simulink model "simulink_2_balloons"  (R2020b)
settings: Solver=VariableStepAuto  StartTime=0.0  StopTime=300  RelTol=1e-3
InitFcn:
  | seed1 = randi(100000);
  | seed2 = randi(200000);
values from neighbouring files (symbols this model uses):
  Cd = 0.185    [sim_1balloon.m]    (also in sim_1balloon_test.m; sim_2balloon.m; sim_2balloon_test.m; sim_4balloon.m)
  coefficient_dragq = [-0.285 -0.20532562963 -0.122209481481 -0.036512 0.0509063703704 0.139185185185 0.227464 0.31488237037 0.400579851852 0.483696 0.56337037037 0.638742518519 ... (72581 elements, 181x401)]    [coefficient_dragq.mat]
  coefficient_sideforceq = [0 -0.0269042962963 -0.0553588148148 -0.084976 -0.115368296296 -0.146148148148 -0.176928 -0.207320296296 -0.236937481481 -0.265392 -0.292296296296 -0.317262814815 ... (72581 elements, 181x401)]    [coefficient_sideforceq.mat]
  mb1 = 3/1000    (= 0.003)    [sim_1balloon.m]    (also in sim_1balloon_test.m; sim_2balloon.m; sim_2balloon_test.m; sim_4balloon.m)
  mb2 = 3/1000    (= 0.003)    [sim_2balloon.m]    (also in sim_2balloon_test.m; sim_4balloon.m; sim_4balloon_test.m)
  nH = optimizableVariable('nH',nHB)    [optimiseB2.m]    (also in optimiseB4.m; sim_1balloon.m = x(2); sim_1balloon_test.m = x(2); sim_2balloon.m = x(2))
  normalScaling = optimizableVariable('normalScaling',normalScalingB)    [optimiseB2.m]    (also in optimiseB4.m; sim_1balloon.m = x(5); sim_1balloon_test.m = x(5); sim_2balloon.m = x(5))
  nS = optimizableVariable('nS',nSB)    [optimiseB2.m]    (also in optimiseB4.m; sim_1balloon.m = x(3); sim_1balloon_test.m = x(3); sim_2balloon.m = x(3))
  nV = optimizableVariable('nV',nVB)    [optimiseB2.m]    (also in optimiseB4.m; sim_1balloon.m = x(1); sim_1balloon_test.m = x(1); sim_2balloon.m = x(1))
  rb = 80/1000    (= 0.08)    [sim_1balloon.m]    (also in sim_1balloon_test.m; sim_2balloon.m; sim_2balloon_test.m; sim_4balloon.m)
  rb1 = 80/1000    (= 0.08)    [sim_1balloon.m]    (also in sim_1balloon_test.m; sim_2balloon.m; sim_2balloon_test.m; sim_4balloon.m)
  rb2 = 80/1000    (= 0.08)    [sim_2balloon.m]    (also in sim_2balloon_test.m; sim_4balloon.m; sim_4balloon_test.m)
  rn = 125/2000    (= 0.0625)    [sim_1balloon.m]    (also in sim_1balloon_test.m; sim_2balloon.m; sim_2balloon_test.m; sim_4balloon.m)
  seedX1 = randi(100000)    [sim_1balloon.m]    (also in sim_1balloon_test.m = x(8); sim_2balloon.m; sim_2balloon_test.m = x(11); sim_4balloon.m)
  seedX2 = randi(100000)    [sim_2balloon.m]    (also in sim_2balloon_test.m = x(14); sim_4balloon.m; sim_4balloon_test.m = x(14))
  seedY1 = randi(100000)    [sim_1balloon.m]    (also in sim_1balloon_test.m = x(9); sim_2balloon.m; sim_2balloon_test.m = x(12); sim_4balloon.m)
  seedY2 = randi(100000)    [sim_2balloon.m]    (also in sim_2balloon_test.m = x(15); sim_4balloon.m; sim_4balloon_test.m = x(15))
  seedZ1 = randi(100000)    [sim_1balloon.m]    (also in sim_1balloon_test.m = x(10); sim_2balloon.m; sim_2balloon_test.m = x(13); sim_4balloon.m)
  seedZ2 = randi(100000)    [sim_2balloon.m]    (also in sim_2balloon_test.m = x(16); sim_4balloon.m; sim_4balloon_test.m = x(16))
  theta = optimizableVariable('theta',thetaB)    [optimiseB2.m]    (also in optimiseB4.m; sim_1balloon.m = x(7); sim_1balloon_test.m = x(7); sim_2balloon.m = x(7))
  V0 = optimizableVariable('V0',V0B)    [optimiseB1.m]    (also in optimiseB2.m; optimiseB4.m; sim_1balloon.m = x(4); sim_1balloon_test.m = x(4))
libraries: nesl_utility x21, sm_lib x12, eeGeneralControl x6
settings Model: Creator=toby  LastModifiedBy=dante
settings ExplorerConfigSet: InternalSimMechanicsExplorerSettings="<ExplorerConfiguration><canonicalview>default</canonicalview><AnimationSetting><BasePlaybackSpeed>1.0</BasePlaybackSpeed><PlaybackSpeedFactor>1.0</PlaybackSpeedFactor></AnimationSetting><TilePanel><TileInfo><Tiles Columns=\"1\" Count=\"1\" Rows=\"1\"><Column Weight=\"1\"/><Row Weight=\"1\"/><Tile Height=\"1\" Width=\"1\" X=\"0\" Y=\"0\"/></Tiles></TileInfo><SceneInfo><SceneViewer><BGColor><R>0.60000002384185791</R><G>0.60000002384185791</G><B>0.60000002384185791</B></BGColor><Camera><DoPerspective>off</DoPerspective><Position><X>-0.0428873579630689797</X><Y>-0.981698513031005859</Y><Z>0.930594914501606474</Z></Position><Center><X>-0.0428873579630689797</X><Y>0.0183014869689941406</Y><Z>0.930594914501606474</Z></Center><Up><X>0</X><Y>-0</Y><Z>1</Z></Up><ViewLimDist>1</ViewLimDist><YLim>0.975489363470708692</YLim><XLim>1.38819640186216242</XLim></Camera></SceneViewer></SceneInfo></TilePanel><MechEditorPanel><Cameras/><GfxPanelCameraMap/><VideoCreator><PlaybackSpeedRatio>1.0</PlaybackSpeedRatio><FrameRate>30</FrameRate><VideoFormat>MPEG-4</VideoFormat><FrameSize>auto</FrameSize></VideoCreator></MechEditorPanel></ExplorerConfiguration>"

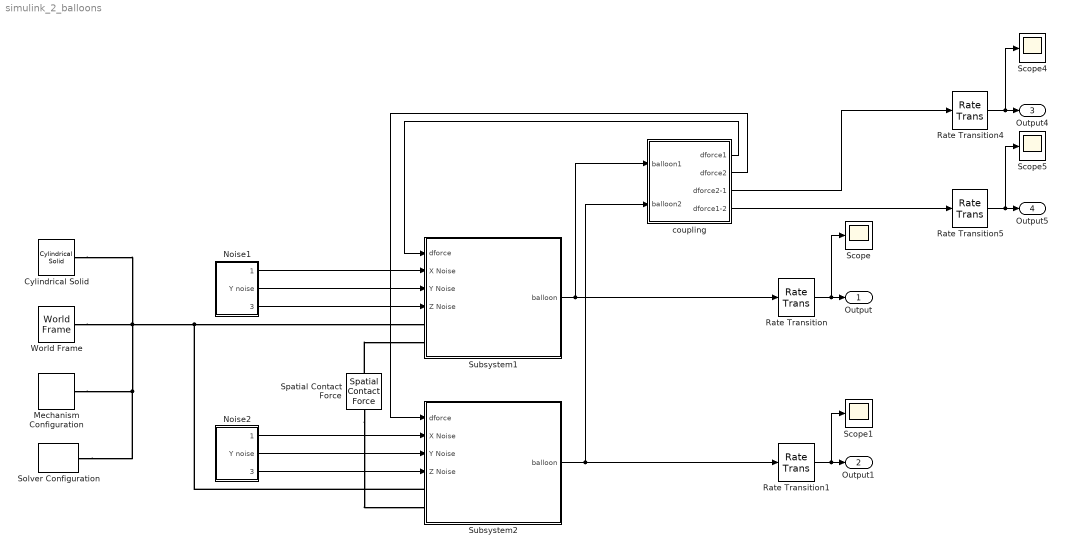
== system simulink_2_balloons ==
  Cylindrical Solid : sm_lib/Body Elements/Cylindrical Solid  GraphicAmbientColor=[0.15 0.15 0.15 1.0]  BasedOnType=Density  CenterOfMass=[0 0 0]  CenterOfMassUnits=m  GraphicDiffuseColor=[0.2 1.0 1.0]  CylinderLength=0.01  CylinderLengthUnits=m  CylinderRadius=rn  CylinderRadiusUnits=m  Density=1000  DensityUnits=kg/m^3  DoExposeReferenceFrame=on  GraphicEmissiveColor=[0.0 0.0 0.0 1.0]  ExportEntireGeometry=off  SerializedFrames=<Frames/>  MarkerShape=Sphere  MarkerSize=10  GraphicType=FromGeometry  InertiaType=CalculateFromGeometry  Mass=1  MassUnits=kg  MomentsOfInertia=[1 1 1]  MomentsOfInertiaUnits=kg*m^2  GraphicOpacity=1.0  ProductsOfInertia=[0 0 0]  ProductsOfInertiaUnits=kg*m^2  GraphicShininess=75  GraphicSpecularColor=[0.5 0.5 0.5 1.0]  GraphicVisPropType=SimpleVisualProperties
  Mechanism Configuration : sm_lib/Utilities/Mechanism Configuration  UniformGravity=Constant  GravityVector=[0 0 -9.81]  GravityVectorUnits=m/s^2  GravityUnits=m/s^2  LinearizationDelta=0.001  JointModeTransitionNonlinearIterations=2
  Noise1 : Subsystem
  Noise2 : Subsystem
  Rate Transition{,1,4..5} (4 alike) : RateTransition  OutPortSampleTime=1/30
  Scope{,1,4..5} (4 alike) : Scope
  Solver Configuration : nesl_utility/Solver Configuration  PhysicalDomain=network_engine_domain  SubClassName=solver  LeftPortType=input  RightPortType=generic  Tones=[]  Harmonics=[]  SimulateNoise=off  Profile=off  UseLocalSampling=off  EnableSwitchedLinearOptims=on  FrequencyDomain=off  UseCCode=off  RelTol=0.001  AbsTol=1e-06  MinStep=1e-09  ToWorkspace=off  RevertToSquareIcSolve=off  NumHomotopyIterations=100  PhasorMode=off  PhasorModeNumHarmonics=1  DoDC=off  ResidualTolerance=1e-9  UseLocalSolver=off  LocalSolverChoice=NE_BACKWARD_EULER_ADVANCER  LocalSolverSampleTime=.001  DoFixedCost=off  MaxNonlinIter=3  MaxModeIter=2  ComputeImpulses=off  ImpulseIterations=2  LinearAlgebra=Sparse  EquationFormulation=NE_TIME_EF  DelaysMemoryBudget=1024  AutomaticFiltering=on  FilteringTimeConstant=0.001  PartitionStorageMethod=AS_NEEDED  PartitionMemoryBudget=1024  PartitionMethod=FAST
  Spatial Contact Force : sm_lib/Forces and Torques/Spatial Contact Force  CoefficientOfDynamicFriction=0.1  CoefficientOfStaticFriction=0.1  NormalDamping=d  NormalDampingUnits=N/(m/s)  NormalStiffness=k  NormalStiffnessUnits=N/m  FrictionalCriticalVelocity=1e-3  FrictionalCriticalVelocityUnits=m/s  ZeroCrossDetectContactStartAndEnd=off  SenseFrictionalForceMagnitude=off  SenseNormalForceMagnitude=off  SenseSeparationDistance=off  NormalTransitionRegionWidth=tw  NormalTransitionRegionWidthUnits=m  FrictionType=SmoothStickSlip
  Subsystem1 : Subsystem  mask{initialHeight=0.2, ix=0, iy=0, balloonRadius=rb1, balloonMass=mb1, nozzleRadius=rn, theta=theta, V0=V0, Cd=Cd, normalScaling=normalScaling}
      mask prompts: initialHeight "initial height"; balloonRadius "balloon radius"; balloonMass "balloon mass"
  Subsystem2 : Subsystem  mask{initialHeight=0.4, ix=0, iy=0, balloonRadius=rb2, balloonMass=mb2, nozzleRadius=rn, theta=theta, V0=V0, Cd=Cd, normalScaling=normalScaling}
      mask prompts: initialHeight "initial height"; balloonRadius "balloon radius"; balloonMass "balloon mass"
  World Frame : sm_lib/Frames and Transforms/World Frame
  coupling : Subsystem
  Output : Outport
  Output1 : Outport  Port=2
  Output4 : Outport  Port=3
  Output5 : Outport  Port=4
  wires:
  Noise1/1(X noise) -> Subsystem1/2(X Noise)
  Rate Transition/1 -> Scope/1, Output/1
  Noise1/3(Z noise) -> Subsystem1/4(Z Noise)
  Noise1/2(" Y noise") -> Subsystem1/3(Y Noise)
  Rate Transition1/1 -> Scope1/1, Output1/1
  Noise2/3(Z noise) -> Subsystem2/4(Z Noise)
  Noise2/2(" Y noise") -> Subsystem2/3(Y Noise)
  Noise2/1(X noise) -> Subsystem2/2(X Noise)
  Subsystem1/1(balloon) -> Rate Transition/1, coupling/1(balloon1)
  coupling/1(dforce1) -> Subsystem1/1(dforce)
  Subsystem2/1(balloon) -> Rate Transition1/1, coupling/2(balloon2)
  coupling/2(dforce2) -> Subsystem2/1(dforce)
  Rate Transition4/1 -> Scope4/1, Output4/1
  Rate Transition5/1 -> Scope5/1, Output5/1
  coupling/3(dforce2-1) -> Rate Transition4/1
  coupling/4(dforce1-2) -> Rate Transition5/1
  connections:
  World Frame/RConn1 -- Solver Configuration/RConn1 -- Mechanism Configuration/RConn1 -- Subsystem2/LConn1 -- Subsystem1/LConn1 -- Cylindrical Solid/RConn1
  Spatial Contact Force/LConn1 -- Subsystem1/LConn2
  Spatial Contact Force/RConn1 -- Subsystem2/LConn2

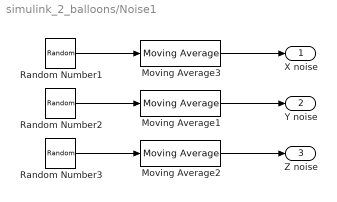
== system simulink_2_balloons/Noise1 ==
  Moving Average1 : eeGeneralControl/Moving Average  VariantControl=Variant1  LabelModeActiveChoice=Discrete  f=10  x0=0  Ts=nS/10
      settings: SourceProductBaseCode=PS
  Moving Average2 : eeGeneralControl/Moving Average  VariantControl=Variant1  LabelModeActiveChoice=Discrete  f=10  x0=0  Ts=nS/10
      settings: SourceProductBaseCode=PS
  Moving Average3 : eeGeneralControl/Moving Average  VariantControl=Variant1  LabelModeActiveChoice=Discrete  f=10  x0=0  Ts=nS/10
      settings: SourceProductBaseCode=PS
  Random Number1 : RandomNumber  Variance=nH  Seed=seedX1  SampleTime=nS
  Random Number2 : RandomNumber  Variance=nH  Seed=seedY1  SampleTime=nS
  Random Number3 : RandomNumber  Variance=nV  Seed=seedZ1  SampleTime=nS
  X noise : Outport
  " Y noise" : Outport  Port=2
  Z noise : Outport  Port=3
  wires:
  Random Number2/1 -> Moving Average1/1
  Moving Average3/1 -> X noise/1
  Random Number3/1 -> Moving Average2/1
  Random Number1/1 -> Moving Average3/1
  Moving Average1/1 -> " Y noise"/1
  Moving Average2/1 -> Z noise/1

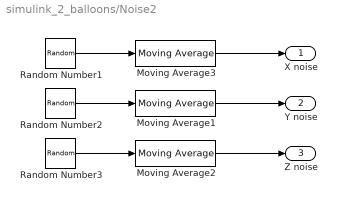
== system simulink_2_balloons/Noise2 ==
  Moving Average1 : eeGeneralControl/Moving Average  VariantControl=Variant1  LabelModeActiveChoice=Discrete  f=10  x0=0  Ts=nS/10
      settings: SourceProductBaseCode=PS
  Moving Average2 : eeGeneralControl/Moving Average  VariantControl=Variant1  LabelModeActiveChoice=Discrete  f=10  x0=0  Ts=nS/10
      settings: SourceProductBaseCode=PS
  Moving Average3 : eeGeneralControl/Moving Average  VariantControl=Variant1  LabelModeActiveChoice=Discrete  f=10  x0=0  Ts=nS/10
      settings: SourceProductBaseCode=PS
  Random Number1 : RandomNumber  Variance=nH  Seed=seedX2  SampleTime=nS
  Random Number2 : RandomNumber  Variance=nH  Seed=seedY2  SampleTime=nS
  Random Number3 : RandomNumber  Variance=nV  Seed=seedZ2  SampleTime=nS
  X noise : Outport
  " Y noise" : Outport  Port=2
  Z noise : Outport  Port=3
  wires:
  Random Number2/1 -> Moving Average1/1
  Moving Average3/1 -> X noise/1
  Random Number3/1 -> Moving Average2/1
  Random Number1/1 -> Moving Average3/1
  Moving Average1/1 -> " Y noise"/1
  Moving Average2/1 -> Z noise/1

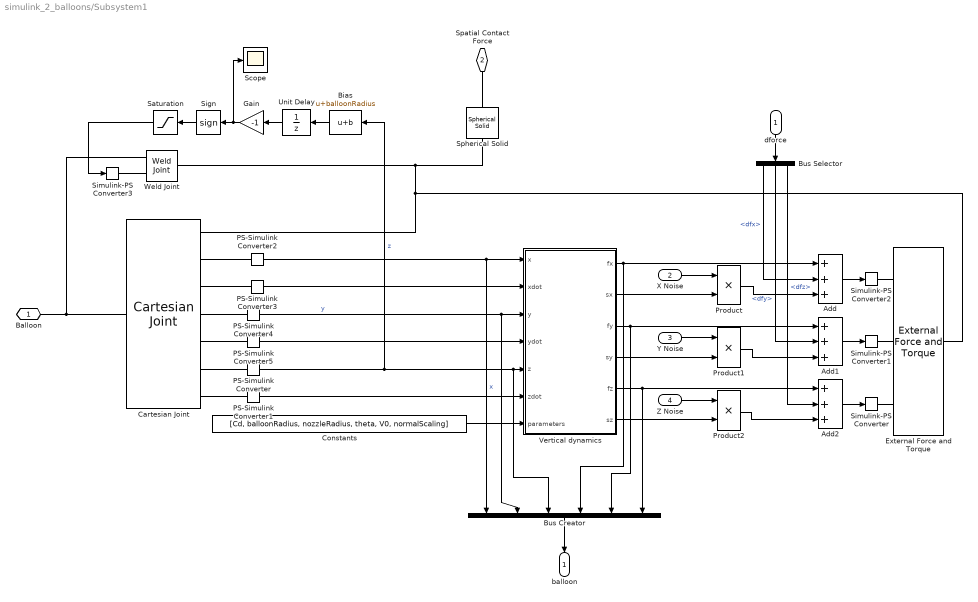
== system simulink_2_balloons/Subsystem1 ==
  dforce : Inport
  X Noise : Inport  Port=2
  Y Noise : Inport  Port=3
  Z Noise : Inport  Port=4
  Add : Sum  Inputs=+++
  Add1 : Sum  Inputs=+++
  Add2 : Sum  Inputs=+++
  Bias : Bias  Bias=balloonRadius
  Bus Creator : BusCreator  Inputs=6
  Bus Selector : BusSelector  OutputSignals=dfx,dfy,dfz
  Cartesian Joint : sm_lib/Joints/Cartesian Joint  JointMode=Normal  SenseConstraintForce=off  SenseConstraintForceX=off  SenseConstraintForceY=off  SenseConstraintForceZ=off  SenseConstraintTorque=off  SenseConstraintTorqueX=off  SenseConstraintTorqueY=off  SenseConstraintTorqueZ=off  SenseTotalForce=off  SenseTotalForceX=off  SenseTotalForceY=off  SenseTotalForceZ=off  SenseTotalTorque=off  SenseTotalTorqueX=off  SenseTotalTorqueY=off  SenseTotalTorqueZ=off  CompositeWrenchDir=FollowerOnBase  CompositeWrenchFrame=BaseFrame  PxEquilibriumPosition=0  PxEquilibriumPositionUnits=m  PxSpringStiffness=0  PxSpringStiffnessUnits=N/m  PxDampingCoefficient=hd  PxDampingCoefficientUnits=N/(m/s)  PxTorqueActuationMode=NoTorque  PxMotionActuationMode=ComputedMotion  PxSensePosition=on  PxSenseVelocity=on  PxSenseAcceleration=off  PxSenseTorqueForce=off  PxSenseLowerLimitTorqueForce=off  PxSenseUpperLimitTorqueForce=off  PxLowerLimitSpecify=off  PxLowerLimitBound=-1  PxLowerLimitBoundUnits=m  PxLowerLimitStiffness=1e6  PxLowerLimitStiffnessUnits=N/m  PxLowerLimitDamping=1e3  PxLowerLimitDampingUnits=N/(m/s)  PxLowerLimitTransitionRegionWidth=1e-4  PxLowerLimitTransitionRegionWidthUnits=m  PxUpperLimitSpecify=off  PxUpperLimitBound=1  PxUpperLimitBoundUnits=m  PxUpperLimitStiffness=1e6  PxUpperLimitStiffnessUnits=N/m  PxUpperLimitDamping=1e3  PxUpperLimitDampingUnits=N/(m/s)  PxUpperLimitTransitionRegionWidth=1e-4  PxUpperLimitTransitionRegionWidthUnits=m  PxPositionTargetSpecify=off  PxPositionTargetPriority=High  PxPositionTargetValue=0  PxPositionTargetValueUnits=m  PxVelocityTargetSpecify=off  PxVelocityTargetPriority=High  PxVelocityTargetValue=0  PxVelocityTargetValueUnits=m/s  PyEquilibriumPosition=0  PyEquilibriumPositionUnits=m  PySpringStiffness=0  PySpringStiffnessUnits=N/m  PyDampingCoefficient=hd  PyDampingCoefficientUnits=N/(m/s)  PyTorqueActuationMode=NoTorque  PyMotionActuationMode=ComputedMotion  PySensePosition=on  PySenseVelocity=on  PySenseAcceleration=off  PySenseTorqueForce=off  PySenseLowerLimitTorqueForce=off  PySenseUpperLimitTorqueForce=off  PyLowerLimitSpecify=off  PyLowerLimitBound=-1  PyLowerLimitBoundUnits=m  PyLowerLimitStiffness=1e6  PyLowerLimitStiffnessUnits=N/m  PyLowerLimitDamping=1e3  PyLowerLimitDampingUnits=N/(m/s)  PyLowerLimitTransitionRegionWidth=1e-4  PyLowerLimitTransitionRegionWidthUnits=m  PyUpperLimitSpecify=off  PyUpperLimitBound=1  PyUpperLimitBoundUnits=m  PyUpperLimitStiffness=1e6  PyUpperLimitStiffnessUnits=N/m  PyUpperLimitDamping=1e3  PyUpperLimitDampingUnits=N/(m/s)  PyUpperLimitTransitionRegionWidth=1e-4  PyUpperLimitTransitionRegionWidthUnits=m  PyPositionTargetSpecify=off  PyPositionTargetPriority=High  PyPositionTargetValue=0  PyPositionTargetValueUnits=m  PyVelocityTargetSpecify=off  PyVelocityTargetPriority=High  PyVelocityTargetValue=0  PyVelocityTargetValueUnits=m/s  PzEquilibriumPosition=0  PzEquilibriumPositionUnits=m  PzSpringStiffness=0  PzSpringStiffnessUnits=N/m  PzDampingCoefficient=hd  PzDampingCoefficientUnits=N/(m/s)  PzTorqueActuationMode=NoTorque  PzMotionActuationMode=ComputedMotion  PzSensePosition=on  PzSenseVelocity=on  PzSenseAcceleration=off  PzSenseTorqueForce=off  PzSenseLowerLimitTorqueForce=off  PzSenseUpperLimitTorqueForce=off  PzLowerLimitSpecify=off  PzLowerLimitBound=0  PzLowerLimitBoundUnits=m  PzLowerLimitStiffness=1e6  PzLowerLimitStiffnessUnits=N/m  PzLowerLimitDamping=1e3  PzLowerLimitDampingUnits=N/(m/s)  PzLowerLimitTransitionRegionWidth=1e-4  PzLowerLimitTransitionRegionWidthUnits=m  PzUpperLimitSpecify=off  PzUpperLimitBound=1  PzUpperLimitBoundUnits=m  PzUpperLimitStiffness=1e6  PzUpperLimitStiffnessUnits=N/m  PzUpperLimitDamping=1e3  PzUpperLimitDampingUnits=N/(m/s)  PzUpperLimitTransitionRegionWidth=1e-4  PzUpperLimitTransitionRegionWidthUnits=m  PzPositionTargetSpecify=on  PzPositionTargetPriority=High  PzPositionTargetValue=initialHeight  PzPositionTargetValueUnits=m  PzVelocityTargetSpecify=on  PzVelocityTargetPriority=High  PzVelocityTargetValue=0  PzVelocityTargetValueUnits=m/s
  Constants : Constant  Value=[Cd, balloonRadius, nozzleRadius, theta, V0, normalScaling]
  External Force and Torque : sm_lib/Forces and Torques/External Force and Torque  ForceResolutionFrame=AttachedFrame  EnableForceX=on  EnableForceY=on  EnableForceZ=on  EnableForce=off  TorqueResolutionFrame=AttachedFrame  EnableTorqueX=off  EnableTorqueY=off  EnableTorqueZ=off  EnableTorque=off
  Gain : Gain  Gain=-1
  PS-Simulink Converter{,1..5} (6 alike) : nesl_utility/PS-Simulink Converter  PhysicalDomain=network_engine_domain  SubClassName=ps_output  LeftPortType=input  RightPortType=output  PseudoPeriodic=off  Frequencies=[]  Unit=inherit  AffineConversion=off
  Product : Product
  Product1 : Product
  Product2 : Product
  Saturation : Saturate  UpperLimit=0  LowerLimit=-1
  Scope : Scope
  Sign : Signum
  Simulink-PS Converter{,1..3} (4 alike) : nesl_utility/Simulink-PS Converter  PhysicalDomain=network_engine_domain  SubClassName=ps_input  LeftPortType=input  RightPortType=output  PseudoPeriodic=off  Frequencies=[]  NoiseDistribution=none  NoiseParameters=[]  Unit=1  AffineConversion=off  FilteringAndDerivatives=provide  SimscapeFilterOrder=1  InputFilterTimeConstant=0.001  UdotUserProvided=0
  Spherical Solid : sm_lib/Body Elements/Spherical Solid  GraphicAmbientColor=[0.15 0.15 0.15 1.0]  BasedOnType=Mass  CenterOfMass=[0 0 0]  CenterOfMassUnits=m  GraphicDiffuseColor=[1.0 0.0 0.0]  Density=1000  DensityUnits=kg/m^3  DoExposeReferenceFrame=on  GraphicEmissiveColor=[0.0 0.0 0.0 1.0]  ExportEntireGeometry=on  SerializedExposedGeometries=<ExposedGeometries><ExposedGeometry><RawGeometryId>entire</RawGeometryId><ExposedGeometryId>G</ExposedGeometryId></ExposedGeometry></ExposedGeometries>  SerializedFrames=<Frames/>  MarkerShape=Sphere  MarkerSize=10  GraphicType=FromGeometry  InertiaType=CalculateFromGeometry  Mass=balloonMass  MassUnits=kg  MomentsOfInertia=[1 1 1]  MomentsOfInertiaUnits=kg*m^2  GraphicOpacity=1.0  ProductsOfInertia=[0 0 0]  ProductsOfInertiaUnits=kg*m^2  GraphicShininess=75  GraphicSpecularColor=[0.5 0.5 0.5 1.0]  SphereRadius=balloonRadius  SphereRadiusUnits=m  GraphicVisPropType=SimpleVisualProperties
  Unit Delay : UnitDelay  InitialCondition=initialHeight+balloonRadius  SampleTime=0.01  HasFrameUpgradeWarning=on
  Vertical dynamics : MATLAB Function  TreatAsAtomicUnit=on
  Weld Joint : sm_lib/Joints/Weld Joint  JointMode=ProvidedByInput  SenseConstraintForce=off  SenseConstraintForceX=off  SenseConstraintForceY=off  SenseConstraintForceZ=off  SenseConstraintTorque=off  SenseConstraintTorqueX=off  SenseConstraintTorqueY=off  SenseConstraintTorqueZ=off  SenseTotalForce=off  SenseTotalForceX=off  SenseTotalForceY=off  SenseTotalForceZ=off  SenseTotalTorque=off  SenseTotalTorqueX=off  SenseTotalTorqueY=off  SenseTotalTorqueZ=off  CompositeWrenchDir=FollowerOnBase  CompositeWrenchFrame=BaseFrame
  Balloon : PMIOPort  Side=Left
  Spatial Contact Force : PMIOPort  Port=2  Side=Left
  balloon : Outport
  wires:
  PS-Simulink Converter3/1 -> Vertical dynamics/2(xdot)
  PS-Simulink Converter4/1 -> Vertical dynamics/3(y), Bus Creator/2  "y"
  PS-Simulink Converter2/1 -> Vertical dynamics/1(x), Bus Creator/1  "x"
  PS-Simulink Converter5/1 -> Vertical dynamics/4(ydot)
  Constants/1 -> Vertical dynamics/7(parameters)
  PS-Simulink Converter/1 -> Bus Creator/3, Vertical dynamics/5(z), Bias/1  "z"
  PS-Simulink Converter1/1 -> Vertical dynamics/6(zdot)
  Vertical dynamics/2(sx) -> Product/2
  Vertical dynamics/4(sy) -> Product1/2
  Vertical dynamics/6(sz) -> Product2/2
  Gain/1 -> Scope/1, Sign/1
  Unit Delay/1 -> Gain/1
  Sign/1 -> Saturation/1
  Saturation/1 -> Simulink-PS Converter3/1
  Bias/1 -> Unit Delay/1
  Z Noise/1 -> Product2/1
  Add/1 -> Simulink-PS Converter2/1
  Add1/1 -> Simulink-PS Converter1/1
  Add2/1 -> Simulink-PS Converter/1
  Y Noise/1 -> Product1/1
  X Noise/1 -> Product/1
  Vertical dynamics/5(fz) -> Add2/1, Bus Creator/6
  Vertical dynamics/3(fy) -> Add1/1, Bus Creator/5
  Vertical dynamics/1(fx) -> Add/1, Bus Creator/4
  Bus Creator/1 -> balloon/1
  dforce/1 -> Bus Selector/1
  Product2/1 -> Add2/3
  Product1/1 -> Add1/3
  Product/1 -> Add/3
  Bus Selector/3 -> Add2/2  "<dfz>"
  Bus Selector/2 -> Add1/2  "<dfy>"
  Bus Selector/1 -> Add/2  "<dfx>"
  connections:
  PS-Simulink Converter/LConn1 -- Cartesian Joint/RConn6
  PS-Simulink Converter2/LConn1 -- Cartesian Joint/RConn2
  Weld Joint/RConn1 -- Spherical Solid/RConn1 -- Cartesian Joint/RConn1 -- External Force and Torque/RConn1
  Cartesian Joint/LConn1 -- Weld Joint/LConn1 -- Balloon/RConn1
  PS-Simulink Converter5/LConn1 -- Cartesian Joint/RConn5
  Simulink-PS Converter/RConn1 -- External Force and Torque/LConn3
  External Force and Torque/LConn1 -- Simulink-PS Converter2/RConn1
  Simulink-PS Converter1/RConn1 -- External Force and Torque/LConn2
  Cartesian Joint/RConn4 -- PS-Simulink Converter4/LConn1
  PS-Simulink Converter3/LConn1 -- Cartesian Joint/RConn3
  PS-Simulink Converter1/LConn1 -- Cartesian Joint/RConn7
  Simulink-PS Converter3/RConn1 -- Weld Joint/LConn2
  Spatial Contact Force/RConn1 -- Spherical Solid/LConn1

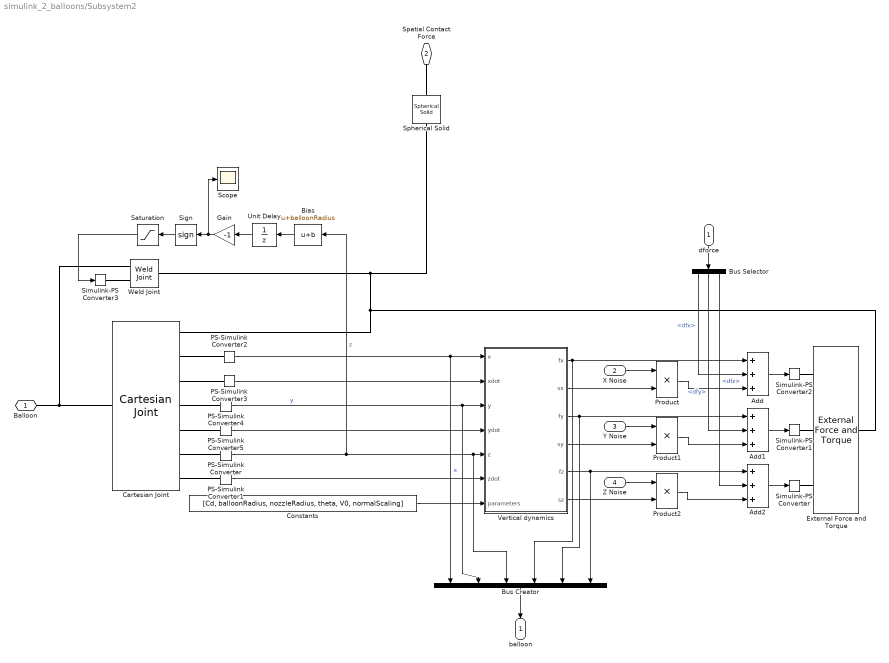
== system simulink_2_balloons/Subsystem2 ==
  dforce : Inport
  X Noise : Inport  Port=2
  Y Noise : Inport  Port=3
  Z Noise : Inport  Port=4
  Add : Sum  Inputs=+++
  Add1 : Sum  Inputs=+++
  Add2 : Sum  Inputs=+++
  Bias : Bias  Bias=balloonRadius
  Bus Creator : BusCreator  Inputs=6
  Bus Selector : BusSelector  OutputSignals=dfx,dfy,dfz
  Cartesian Joint : sm_lib/Joints/Cartesian Joint  JointMode=Normal  SenseConstraintForce=off  SenseConstraintForceX=off  SenseConstraintForceY=off  SenseConstraintForceZ=off  SenseConstraintTorque=off  SenseConstraintTorqueX=off  SenseConstraintTorqueY=off  SenseConstraintTorqueZ=off  SenseTotalForce=off  SenseTotalForceX=off  SenseTotalForceY=off  SenseTotalForceZ=off  SenseTotalTorque=off  SenseTotalTorqueX=off  SenseTotalTorqueY=off  SenseTotalTorqueZ=off  CompositeWrenchDir=FollowerOnBase  CompositeWrenchFrame=BaseFrame  PxEquilibriumPosition=0  PxEquilibriumPositionUnits=m  PxSpringStiffness=0  PxSpringStiffnessUnits=N/m  PxDampingCoefficient=hd  PxDampingCoefficientUnits=N/(m/s)  PxTorqueActuationMode=NoTorque  PxMotionActuationMode=ComputedMotion  PxSensePosition=on  PxSenseVelocity=on  PxSenseAcceleration=off  PxSenseTorqueForce=off  PxSenseLowerLimitTorqueForce=off  PxSenseUpperLimitTorqueForce=off  PxLowerLimitSpecify=off  PxLowerLimitBound=-1  PxLowerLimitBoundUnits=m  PxLowerLimitStiffness=1e6  PxLowerLimitStiffnessUnits=N/m  PxLowerLimitDamping=1e3  PxLowerLimitDampingUnits=N/(m/s)  PxLowerLimitTransitionRegionWidth=1e-4  PxLowerLimitTransitionRegionWidthUnits=m  PxUpperLimitSpecify=off  PxUpperLimitBound=1  PxUpperLimitBoundUnits=m  PxUpperLimitStiffness=1e6  PxUpperLimitStiffnessUnits=N/m  PxUpperLimitDamping=1e3  PxUpperLimitDampingUnits=N/(m/s)  PxUpperLimitTransitionRegionWidth=1e-4  PxUpperLimitTransitionRegionWidthUnits=m  PxPositionTargetSpecify=off  PxPositionTargetPriority=High  PxPositionTargetValue=0  PxPositionTargetValueUnits=m  PxVelocityTargetSpecify=off  PxVelocityTargetPriority=High  PxVelocityTargetValue=0  PxVelocityTargetValueUnits=m/s  PyEquilibriumPosition=0  PyEquilibriumPositionUnits=m  PySpringStiffness=0  PySpringStiffnessUnits=N/m  PyDampingCoefficient=hd  PyDampingCoefficientUnits=N/(m/s)  PyTorqueActuationMode=NoTorque  PyMotionActuationMode=ComputedMotion  PySensePosition=on  PySenseVelocity=on  PySenseAcceleration=off  PySenseTorqueForce=off  PySenseLowerLimitTorqueForce=off  PySenseUpperLimitTorqueForce=off  PyLowerLimitSpecify=off  PyLowerLimitBound=-1  PyLowerLimitBoundUnits=m  PyLowerLimitStiffness=1e6  PyLowerLimitStiffnessUnits=N/m  PyLowerLimitDamping=1e3  PyLowerLimitDampingUnits=N/(m/s)  PyLowerLimitTransitionRegionWidth=1e-4  PyLowerLimitTransitionRegionWidthUnits=m  PyUpperLimitSpecify=off  PyUpperLimitBound=1  PyUpperLimitBoundUnits=m  PyUpperLimitStiffness=1e6  PyUpperLimitStiffnessUnits=N/m  PyUpperLimitDamping=1e3  PyUpperLimitDampingUnits=N/(m/s)  PyUpperLimitTransitionRegionWidth=1e-4  PyUpperLimitTransitionRegionWidthUnits=m  PyPositionTargetSpecify=off  PyPositionTargetPriority=High  PyPositionTargetValue=0  PyPositionTargetValueUnits=m  PyVelocityTargetSpecify=off  PyVelocityTargetPriority=High  PyVelocityTargetValue=0  PyVelocityTargetValueUnits=m/s  PzEquilibriumPosition=0  PzEquilibriumPositionUnits=m  PzSpringStiffness=0  PzSpringStiffnessUnits=N/m  PzDampingCoefficient=hd  PzDampingCoefficientUnits=N/(m/s)  PzTorqueActuationMode=NoTorque  PzMotionActuationMode=ComputedMotion  PzSensePosition=on  PzSenseVelocity=on  PzSenseAcceleration=off  PzSenseTorqueForce=off  PzSenseLowerLimitTorqueForce=off  PzSenseUpperLimitTorqueForce=off  PzLowerLimitSpecify=off  PzLowerLimitBound=0  PzLowerLimitBoundUnits=m  PzLowerLimitStiffness=1e6  PzLowerLimitStiffnessUnits=N/m  PzLowerLimitDamping=1e3  PzLowerLimitDampingUnits=N/(m/s)  PzLowerLimitTransitionRegionWidth=1e-4  PzLowerLimitTransitionRegionWidthUnits=m  PzUpperLimitSpecify=off  PzUpperLimitBound=1  PzUpperLimitBoundUnits=m  PzUpperLimitStiffness=1e6  PzUpperLimitStiffnessUnits=N/m  PzUpperLimitDamping=1e3  PzUpperLimitDampingUnits=N/(m/s)  PzUpperLimitTransitionRegionWidth=1e-4  PzUpperLimitTransitionRegionWidthUnits=m  PzPositionTargetSpecify=on  PzPositionTargetPriority=High  PzPositionTargetValue=initialHeight  PzPositionTargetValueUnits=m  PzVelocityTargetSpecify=on  PzVelocityTargetPriority=High  PzVelocityTargetValue=0  PzVelocityTargetValueUnits=m/s
  Constants : Constant  Value=[Cd, balloonRadius, nozzleRadius, theta, V0, normalScaling]
  External Force and Torque : sm_lib/Forces and Torques/External Force and Torque  ForceResolutionFrame=AttachedFrame  EnableForceX=on  EnableForceY=on  EnableForceZ=on  EnableForce=off  TorqueResolutionFrame=AttachedFrame  EnableTorqueX=off  EnableTorqueY=off  EnableTorqueZ=off  EnableTorque=off
  Gain : Gain  Gain=-1
  PS-Simulink Converter{,1..5} (6 alike) : nesl_utility/PS-Simulink Converter  PhysicalDomain=network_engine_domain  SubClassName=ps_output  LeftPortType=input  RightPortType=output  PseudoPeriodic=off  Frequencies=[]  Unit=inherit  AffineConversion=off
  Product : Product
  Product1 : Product
  Product2 : Product
  Saturation : Saturate  UpperLimit=0  LowerLimit=-1
  Scope : Scope
  Sign : Signum
  Simulink-PS Converter{,1..3} (4 alike) : nesl_utility/Simulink-PS Converter  PhysicalDomain=network_engine_domain  SubClassName=ps_input  LeftPortType=input  RightPortType=output  PseudoPeriodic=off  Frequencies=[]  NoiseDistribution=none  NoiseParameters=[]  Unit=1  AffineConversion=off  FilteringAndDerivatives=provide  SimscapeFilterOrder=1  InputFilterTimeConstant=0.001  UdotUserProvided=0
  Spherical Solid : sm_lib/Body Elements/Spherical Solid  GraphicAmbientColor=[0.15 0.15 0.15 1.0]  BasedOnType=Mass  CenterOfMass=[0 0 0]  CenterOfMassUnits=m  GraphicDiffuseColor=[0.0 1.0 0.0]  Density=1000  DensityUnits=kg/m^3  DoExposeReferenceFrame=on  GraphicEmissiveColor=[0.0 0.0 0.0 1.0]  ExportEntireGeometry=on  SerializedExposedGeometries=<ExposedGeometries><ExposedGeometry><RawGeometryId>entire</RawGeometryId><ExposedGeometryId>G</ExposedGeometryId></ExposedGeometry></ExposedGeometries>  SerializedFrames=<Frames/>  MarkerShape=Sphere  MarkerSize=10  GraphicType=FromGeometry  InertiaType=CalculateFromGeometry  Mass=balloonMass  MassUnits=kg  MomentsOfInertia=[1 1 1]  MomentsOfInertiaUnits=kg*m^2  GraphicOpacity=1.0  ProductsOfInertia=[0 0 0]  ProductsOfInertiaUnits=kg*m^2  GraphicShininess=75  GraphicSpecularColor=[0.5 0.5 0.5 1.0]  SphereRadius=balloonRadius  SphereRadiusUnits=m  GraphicVisPropType=SimpleVisualProperties
  Unit Delay : UnitDelay  InitialCondition=initialHeight+balloonRadius  SampleTime=0.01  HasFrameUpgradeWarning=on
  Vertical dynamics : MATLAB Function  TreatAsAtomicUnit=on
  Weld Joint : sm_lib/Joints/Weld Joint  JointMode=ProvidedByInput  SenseConstraintForce=off  SenseConstraintForceX=off  SenseConstraintForceY=off  SenseConstraintForceZ=off  SenseConstraintTorque=off  SenseConstraintTorqueX=off  SenseConstraintTorqueY=off  SenseConstraintTorqueZ=off  SenseTotalForce=off  SenseTotalForceX=off  SenseTotalForceY=off  SenseTotalForceZ=off  SenseTotalTorque=off  SenseTotalTorqueX=off  SenseTotalTorqueY=off  SenseTotalTorqueZ=off  CompositeWrenchDir=FollowerOnBase  CompositeWrenchFrame=BaseFrame
  Balloon : PMIOPort  Side=Left
  Spatial Contact Force : PMIOPort  Port=2  Side=Left
  balloon : Outport
  wires:
  PS-Simulink Converter4/1 -> Vertical dynamics/3(y), Bus Creator/2  "y"
  PS-Simulink Converter2/1 -> Bus Creator/1, Vertical dynamics/1(x)  "x"
  Gain/1 -> Scope/1, Sign/1
  Unit Delay/1 -> Gain/1
  Sign/1 -> Saturation/1
  Saturation/1 -> Simulink-PS Converter3/1
  Bias/1 -> Unit Delay/1
  Product2/1 -> Add2/3
  Bus Selector/2 -> Add1/2  "<dfy>"
  Bus Selector/3 -> Add2/2  "<dfz>"
  Vertical dynamics/1(fx) -> Add/1, Bus Creator/4
  Vertical dynamics/5(fz) -> Add2/1, Bus Creator/6
  PS-Simulink Converter/1 -> Bus Creator/3, Vertical dynamics/5(z), Bias/1  "z"
  X Noise/1 -> Product/1
  Vertical dynamics/4(sy) -> Product1/2
  Add1/1 -> Simulink-PS Converter1/1
  Add/1 -> Simulink-PS Converter2/1
  Add2/1 -> Simulink-PS Converter/1
  Vertical dynamics/3(fy) -> Add1/1, Bus Creator/5
  Y Noise/1 -> Product1/1
  Vertical dynamics/2(sx) -> Product/2
  Product1/1 -> Add1/3
  Product/1 -> Add/3
  dforce/1 -> Bus Selector/1
  Vertical dynamics/6(sz) -> Product2/2
  Bus Creator/1 -> balloon/1
  Z Noise/1 -> Product2/1
  Bus Selector/1 -> Add/2  "<dfx>"
  PS-Simulink Converter5/1 -> Vertical dynamics/4(ydot)
  PS-Simulink Converter1/1 -> Vertical dynamics/6(zdot)
  PS-Simulink Converter3/1 -> Vertical dynamics/2(xdot)
  Constants/1 -> Vertical dynamics/7(parameters)
  connections:
  PS-Simulink Converter/LConn1 -- Cartesian Joint/RConn6
  PS-Simulink Converter2/LConn1 -- Cartesian Joint/RConn2
  Weld Joint/RConn1 -- Spherical Solid/RConn1 -- External Force and Torque/RConn1 -- Cartesian Joint/RConn1
  Cartesian Joint/LConn1 -- Weld Joint/LConn1 -- Balloon/RConn1
  PS-Simulink Converter5/LConn1 -- Cartesian Joint/RConn5
  Cartesian Joint/RConn4 -- PS-Simulink Converter4/LConn1
  PS-Simulink Converter3/LConn1 -- Cartesian Joint/RConn3
  PS-Simulink Converter1/LConn1 -- Cartesian Joint/RConn7
  Simulink-PS Converter3/RConn1 -- Weld Joint/LConn2
  Spatial Contact Force/RConn1 -- Spherical Solid/LConn1
  Simulink-PS Converter1/RConn1 -- External Force and Torque/LConn2
  Simulink-PS Converter/RConn1 -- External Force and Torque/LConn3
  External Force and Torque/LConn1 -- Simulink-PS Converter2/RConn1

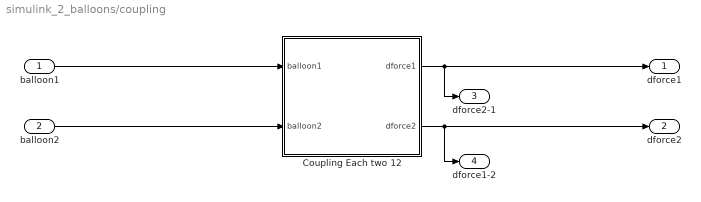
== system simulink_2_balloons/coupling ==
  balloon1 : Inport
  balloon2 : Inport  Port=2
  Coupling Each two 12 : Subsystem
  dforce1 : Outport
  dforce2 : Outport  Port=2
  dforce2-1 : Outport  Port=3
  dforce1-2 : Outport  Port=4
  wires:
  balloon1/1 -> Coupling Each two 12/1(balloon1)
  balloon2/1 -> Coupling Each two 12/2(balloon2)
  Coupling Each two 12/1(dforce1) -> dforce1/1, dforce2-1/1
  Coupling Each two 12/2(dforce2) -> dforce1-2/1, dforce2/1

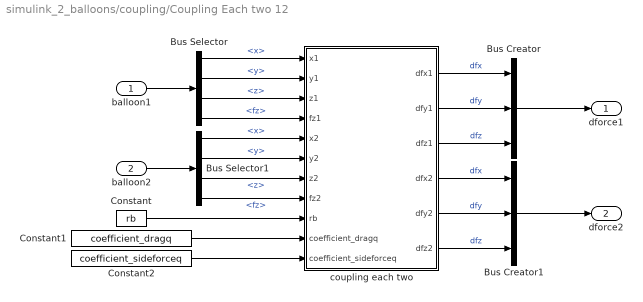
== system simulink_2_balloons/coupling/Coupling Each two 12 ==
  balloon1 : Inport
  balloon2 : Inport  Port=2
  Bus Creator : BusCreator  Inputs=3
  Bus Creator1 : BusCreator  Inputs=3
  Bus Selector : BusSelector  OutputSignals=x,y,z,fz
  Bus Selector1 : BusSelector  OutputSignals=x,y,z,fz
  Constant : Constant  Value=rb
  Constant1 : Constant  Value=coefficient_dragq
  Constant2 : Constant  Value=coefficient_sideforceq
  coupling each two : MATLAB Function  TreatAsAtomicUnit=on
  dforce1 : Outport
  dforce2 : Outport  Port=2
  wires:
  coupling each two/3(dfz1) -> Bus Creator/3  "dfz"
  coupling each two/2(dfy1) -> Bus Creator/2  "dfy"
  coupling each two/1(dfx1) -> Bus Creator/1  "dfx"
  Bus Creator/1 -> dforce1/1
  coupling each two/4(dfx2) -> Bus Creator1/1  "dfx"
  coupling each two/5(dfy2) -> Bus Creator1/2  "dfy"
  coupling each two/6(dfz2) -> Bus Creator1/3  "dfz"
  Bus Creator1/1 -> dforce2/1
  balloon1/1 -> Bus Selector/1
  Bus Selector/4 -> coupling each two/4(fz1)  "<fz>"
  Bus Selector/1 -> coupling each two/1(x1)  "<x>"
  Bus Selector/2 -> coupling each two/2(y1)  "<y>"
  Bus Selector/3 -> coupling each two/3(z1)  "<z>"
  balloon2/1 -> Bus Selector1/1
  Bus Selector1/1 -> coupling each two/5(x2)  "<x>"
  Bus Selector1/2 -> coupling each two/6(y2)  "<y>"
  Bus Selector1/3 -> coupling each two/7(z2)  "<z>"
  Bus Selector1/4 -> coupling each two/8(fz2)  "<fz>"
  Constant/1 -> coupling each two/9(rb)
  Constant1/1 -> coupling each two/10(coefficient_dragq)
  Constant2/1 -> coupling each two/11(coefficient_sideforceq)

== matlab function simulink_2_balloons/Subsystem2/Vertical dynamics ==
  data: fx output; sx output; fy output; sy output; x input; xdot input; y input; ydot input; z input; fz output; zdot input; parameters input; sz output
function [fx,sx,fy,sy,fz,sz] = fcn(x,xdot,y,ydot,z,zdot,parameters)

Cd = parameters(1);
rb = parameters(2);
rn = parameters(3);
theta = deg2rad(parameters(4)); 
V0 = parameters(5); 
normalScaling = parameters(6); 

%% Vertical forces

%flow radius
rFlow = rn+z*tan(theta);

%Peak flow velocity
meanFlowVelocity = V0*rn^2/(rFlow)^2;

%Velocity under ball
vFlowActual = flowSpeed(meanFlowVelocity,normalScaling*rFlow,x,y);

%Relative
relativeVelocity = vFlowActual - zdot;

%Force
fz = sign(relativeVelocity)*0.5*Cd*pi*rb^2*1.22*relativeVelocity^2;



%% Horizontal XY forces
% Bernoulli's Principle
if x == 0 && y == 0
    fx = 0;
    fy = 0;
else
    direction = [x y];
    distance = norm(direction);
    one_direction = direction/distance;
    inner_position = (distance - rb)*one_direction;
    outer_position = (distance + rb)*one_direction;
    vInner = flowSpeed(meanFlowVelocity,normalScaling*rFlow,inner_position(1),inner_position(2));
    vOuter = flowSpeed(meanFlowVelocity,normalScaling*rFlow,outer_position(1),outer_position(2));
    fH = 0.5*1.22*(vOuter^2 - vInner^2)*pi*rb^2*one_direction;
    fx = fH(1);
    fy = fH(2);
end
% Drag
if xdot == 0 && ydot == 0
else
    vxy = [xdot ydot];
    dragH = 0.5*Cd*pi*rb^2*1.22*(xdot^2 + ydot^2)*vxy/norm(vxy);
    fx = fx - dragH(1);
    fy = fy - dragH(2);
end

%% Force scalings
sx = flowSpeed(meanFlowVelocity,normalScaling*rFlow,x,0)/flowSpeed(meanFlowVelocity,rFlow,0,0);
sy = flowSpeed(meanFlowVelocity,normalScaling*rFlow,0,y)/flowSpeed(meanFlowVelocity,rFlow,0,0);
sz = flowSpeed(meanFlowVelocity,normalScaling*rFlow,x,y)/flowSpeed(meanFlowVelocity,rFlow,0,0);

== matlab function simulink_2_balloons/Subsystem1/Vertical dynamics ==
  data: fx output; sx output; fy output; sy output; x input; xdot input; y input; ydot input; z input; fz output; zdot input; parameters input; sz output
function [fx,sx,fy,sy,fz,sz] = fcn(x,xdot,y,ydot,z,zdot,parameters)

Cd = parameters(1);
rb = parameters(2);
rn = parameters(3);
theta = deg2rad(parameters(4)); 
V0 = parameters(5); 
normalScaling = parameters(6); 

%% Vertical forces

%flow radius
rFlow = rn+z*tan(theta);

%Peak flow velocity
meanFlowVelocity = V0*rn^2/(rFlow)^2;

%Velocity under ball
vFlowActual = flowSpeed(meanFlowVelocity,normalScaling*rFlow,x,y);

%Relative
relativeVelocity = vFlowActual - zdot;

%Force
fz = sign(relativeVelocity)*0.5*Cd*pi*rb^2*1.22*relativeVelocity^2;



%% Horizontal XY forces
% Bernoulli's Principle
if x == 0 && y == 0
    fx = 0;
    fy = 0;
else
    direction = [x y];
    distance = norm(direction);
    one_direction = direction/distance;
    inner_position = (distance - rb)*one_direction;
    outer_position = (distance + rb)*one_direction;
    vInner = flowSpeed(meanFlowVelocity,normalScaling*rFlow,inner_position(1),inner_position(2));
    vOuter = flowSpeed(meanFlowVelocity,normalScaling*rFlow,outer_position(1),outer_position(2));
    fH = 0.5*1.22*(vOuter^2 - vInner^2)*pi*rb^2*one_direction;
    fx = fH(1);
    fy = fH(2);
end
% Drag
if xdot == 0 && ydot == 0
else
    vxy = [xdot ydot];
    dragH = 0.5*Cd*pi*rb^2*1.22*(xdot^2 + ydot^2)*vxy/norm(vxy);
    fx = fx - dragH(1);
    fy = fy - dragH(2);
end

%% Force scalings
sx = flowSpeed(meanFlowVelocity,normalScaling*rFlow,x,0)/flowSpeed(meanFlowVelocity,rFlow,0,0);
sy = flowSpeed(meanFlowVelocity,normalScaling*rFlow,0,y)/flowSpeed(meanFlowVelocity,rFlow,0,0);
sz = flowSpeed(meanFlowVelocity,normalScaling*rFlow,x,y)/flowSpeed(meanFlowVelocity,rFlow,0,0);

== matlab function simulink_2_balloons/coupling/Coupling Each two 12/coupling each two ==
  data: x1 input; dfx1 output; y1 input; dfy1 output; dfz1 output; dfx2 output; dfy2 output; dfz2 output; z1 input; fz1 input; x2 input; y2 input; z2 input; fz2 input; rb input; coefficient_dragq input; coefficient_sideforceq input
function [dfx1,dfy1,dfz1,dfx2,dfy2,dfz2] = fcn(x1, y1, z1, fz1, x2, y2, z2, fz2, rb, coefficient_dragq, coefficient_sideforceq)
    % set vector between balloons and z axis
    vector = [x2-x1 y2-y1 z2-z1];
    vectorz = [0 0 1];
    % distance of balloons
    R = norm(vector)/rb/2;
    
    if R >5 || R < 1 % too far
        dfx1 = 0;
        dfy1 = 0;
        dfz1 = 0;
        dfx2 = 0;
        dfy2 = 0;
        dfz2 = 0;
    else % fit curves
        theta2 = acos(dot(vector,vectorz)/(norm(vector)*norm(vectorz)))/pi*180;
        theta1 = 180 - theta2;
        hvector2 = [x2-x1 y2-y1];
        hvector1 = [x1-x2 y1-y2];
        thetaq1 = floor((theta1-0)/1) + 1;
        thetaq2 = floor((theta2-0)/1) + 1;
        Rq1 = floor((R-1)/0.01) + 1;
        Rq2 = floor((R-1)/0.01) + 1;

        % drag fit
        dfz1 = (coefficient_dragq(thetaq1, Rq1) - 1)*fz1;
        dfz2 = (coefficient_dragq(thetaq2, Rq2) - 1)*fz2;

        % sideforce fit
        if norm(hvector1) == 0 % no sideforce
            dfx1 = 0;
            dfy1 = 0;
            dfx2 = 0;
            dfy2 = 0;
        else
            dsideforce1 = coefficient_sideforceq(thetaq1, Rq1)*fz1*hvector1/norm(hvector1);
            dsideforce2 = coefficient_sideforceq(thetaq2, Rq2)*fz2*hvector2/norm(hvector2);
            dfx1 = dsideforce1(1);
            dfy1 = dsideforce1(2);
            dfx2 = dsideforce2(1);
            dfy2 = dsideforce2(2);
        end
    end
end
